simulink model "preLookupTestGen15"  (R2017b)
settings: Solver=FixedStepDiscrete  StartTime=0.0  StopTime=10.0  RelTol=1e-3
settings Model: Creator=ktrinh  LastModifiedBy=ktrinh
settings DebuggingCC: ParameterOverflowMsg=none

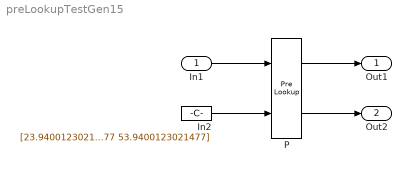
== system preLookupTestGen15 ==
  In1 : Inport  OutDataTypeStr=single  PortDimensions=1
  In2 : Constant  Value=[23.9400123021477 25.4400123021477 26.9400123021477 28.4400123021477 29.9400123021477 31.4400123021477 32.9400123021477 34.4400123021477 35.9400123021477 37.4400123021477 38.9400123021477 40.4400123021477 41.9400123021477 43.4400123021477 44.9400123021477 46.4400123021477 47.9400123021477 49.4400123021477 50.9400123021477 52.4400123021477 53.9400123021477]
  P : PreLookup  BreakpointsDataSource=Input port  BreakpointsData=[10:10:110]  UseLastBreakpoint=on  BreakpointDataTypeStr=uint8  IndexDataTypeStr=uint16  FractionDataTypeStr=single  RndMeth=Convergent
      settings: InputPortMap=u0,p1
  Out1 : Outport
  Out2 : Outport  Port=2
  wires:
  In1/1 -> P/1
  In2/1 -> P/2
  P/1 -> Out1/1
  P/2 -> Out2/1
